simulink model "Lazoabierto_ruido"  (R2021b)
settings: Solver=VariableStepAuto  StartTime=0.0  StopTime=500  RelTol=1e-3
libraries: fl_lib x15, nesl_utility x9, simulink x3, sh_lib x3
settings Model: Creator=sebas  LastModifiedBy=sebas

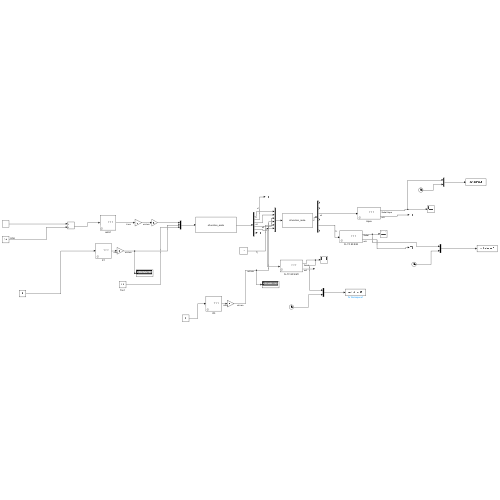
[thumbnail: Simulink's stored preview of the top-level diagram]
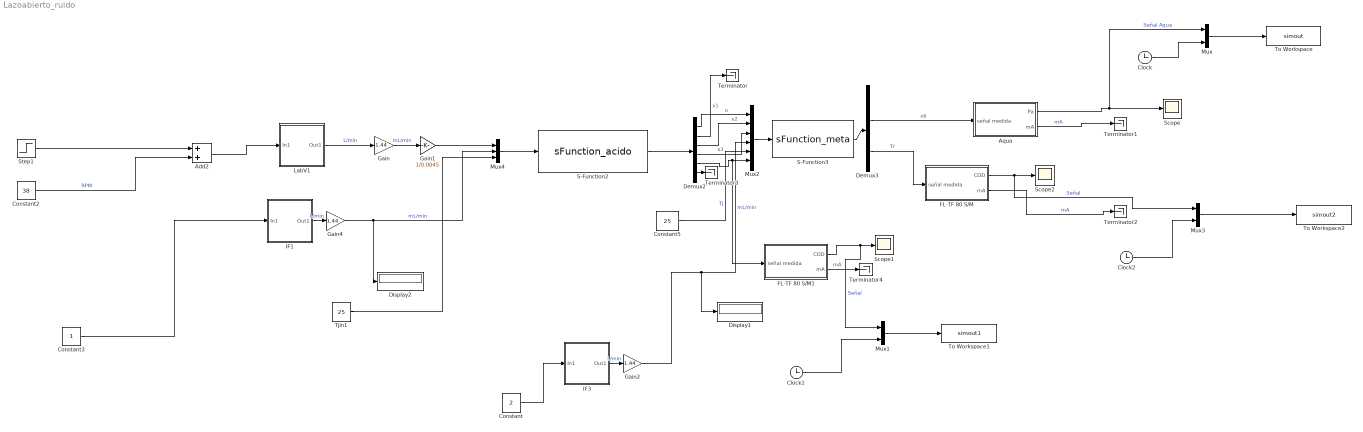
== system Lazoabierto_ruido ==
  Add2 : Sum
  Aqua : Subsystem  mask{To=0.01, d=0, DS=2.5, Ks=0.0056, Tau=1, yo=0, Vi=10}
      mask prompts: To "Tiempo de muestreo (s)"; d "Retardo (s)"; DS "Desviacion estandar (mg/L)"; Ks "Sensibilidad (mA/mg/L)"; Tau "Constante de tiempo (s)"; yo "Sesgo (mg/L)"; Vi "Valor inicial (mg/L)"
      mask init:
      | NP=To*DS*DS;
      mask Display: image(imread('sensor3.png'))
  Clock : Clock
  Clock1 : Clock
  Clock2 : Clock
  Constant : Constant  Value=2
  Constant2 : Constant  Value=38
  Constant3 : Constant
  Constant5 : Constant  Value=25
  Demux2 : Demux  Outputs=6
  Demux3 : Demux  Outputs=6
  Display1 : Display
  Display2 : Display
  FL-TF 80 S/M : Subsystem  mask{To=0.001, d=0, DS=0.15, Ks=0.175, Tau=0.0000667, yo=0, Vi=65}
      mask prompts: To "Tiempo de muestreo (s)"; d "Retardo (s)"; DS "Desviacion estandar (C°)"; Ks "Sensibilidad (mA/C°)"; Tau "Constante de tiempo (s)"; yo "Sesgo (C°)"; Vi "Valor inicial (C°)"
      mask init:
      | NP=To*DS*DS;
      mask Display: image(imread('sensor5.png'))
  FL-TF 80 S/M1 : Subsystem  mask{To=0.001, d=0, DS=0.15, Ks=0.175, Tau=0.0000667, yo=0, Vi=37}
      mask prompts: To "Tiempo de muestreo (s)"; d "Retardo (s)"; DS "Desviacion estandar (C°)"; Ks "Sensibilidad (mA/C°)"; Tau "Constante de tiempo (s)"; yo "Sesgo (C°)"; Vi "Valor inicial (C°)"
      mask init:
      | NP=To*DS*DS;
      mask Display: image(imread('sensor5.png'))
  Gain : Gain  Gain=1.44
  Gain1 : Gain  Gain=1/0.0045
  Gain2 : Gain  Gain=1.44
  Gain4 : Gain  Gain=1.44
  IF1 : Subsystem  mask{D=0.00955414, MaxRPM=350, MaxLPM=4.34, OutP=0.1, FluidDens=997, KinemVisc=0.893e-6, BulkMod=2.2e+9}
      mask prompts: D "Displacement [L/rev]"; MaxRPM "RPM Máximas [RPM]"; MaxLPM "Caudal Máximo [L/min]"; OutP "Presión de Salida [MPa]"; FluidDens "Densidad del Fluido [kg/m^3]"; KinemVisc "Viscosidad Cinemática del Fluido [m^2/s]"; BulkMod "Modulo de Compresibilidad del Fluido [Pa]"
      mask help:
      | Simulación de una Bomba Peristáltica utilizando el paquete Simscape (puede entrar en el subsistema para ver en base a que bloques se construyó).
      |
      | El principal parámetro es el Displacement, que representa cuánto aumenta el flujo de la bomba medido en Litros por Minuto [L/min] según el aumento unitario de Revoluciones por Minuto [RPM].
      |
      | El input de este bloque es una fuente de revoluciones en unidades de RPM, el cual entrega un output de caudal en L/min.
      |
      | El valor del Displacement no puede superar su valor máximo según los parámetros entregados de la bomba.
      mask Display:
      | image('bomba3.png'); % Use "Edit Image" on toolstrip to change.
      | % Bloque creado por Tomás Pröschle Donoso - DCP 2020-2
  IF3 : Subsystem  mask{D=0.00955414, MaxRPM=350, MaxLPM=4.34, OutP=0.1, FluidDens=997, KinemVisc=0.893e-6, BulkMod=2.2e+9}
      mask prompts: D "Displacement [L/rev]"; MaxRPM "RPM Máximas [RPM]"; MaxLPM "Caudal Máximo [L/min]"; OutP "Presión de Salida [MPa]"; FluidDens "Densidad del Fluido [kg/m^3]"; KinemVisc "Viscosidad Cinemática del Fluido [m^2/s]"; BulkMod "Modulo de Compresibilidad del Fluido [Pa]"
      mask help:
      | Simulación de una Bomba Peristáltica utilizando el paquete Simscape (puede entrar en el subsistema para ver en base a que bloques se construyó).
      |
      | El principal parámetro es el Displacement, que representa cuánto aumenta el flujo de la bomba medido en Litros por Minuto [L/min] según el aumento unitario de Revoluciones por Minuto [RPM].
      |
      | El input de este bloque es una fuente de revoluciones en unidades de RPM, el cual entrega un output de caudal en L/min.
      |
      | El valor del Displacement no puede superar su valor máximo según los parámetros entregados de la bomba.
      mask Display:
      | image('bomba3.png'); % Use "Edit Image" on toolstrip to change.
      | % Bloque creado por Tomás Pröschle Donoso - DCP 2020-2
  LabV1 : Subsystem  mask{D=0.00001333, MaxRPM=150, MaxLPM=0.57, OutP=0.1, FluidDens=997, KinemVisc=0.893e-6, BulkMod=2.2e+9}
      mask prompts: D "Displacement [L/rev]"; MaxRPM "RPM Máximas [RPM]"; MaxLPM "Caudal Máximo [L/min]"; OutP "Presión de Salida [MPa]"; FluidDens "Densidad del Fluido [kg/m^3]"; KinemVisc "Viscosidad Cinemática del Fluido [m^2/s]"; BulkMod "Modulo de Compresibilidad del Fluido [Pa]"
      mask help:
      | Simulación de una Bomba Peristáltica utilizando el paquete Simscape (puede entrar en el subsistema para ver en base a que bloques se construyó).
      |
      | El principal parámetro es el Displacement, que representa cuánto aumenta el flujo de la bomba medido en Litros por Minuto [L/min] según el aumento unitario de Revoluciones por Minuto [RPM].
      |
      | El input de este bloque es una fuente de revoluciones en unidades de RPM, el cual entrega un output de caudal en L/min.
      |
      | El valor del Displacement no puede superar su valor máximo según los parámetros entregados de la bomba.
      mask Display:
      | image('bomba1.png'); % Use "Edit Image" on toolstrip to change.
      | % Bloque creado por Tomás Pröschle Donoso - DCP 2020-2
  Mux : Mux  Inputs=2
  Mux1 : Mux  Inputs=2
  Mux2 : Mux  Inputs=6
  Mux3 : Mux  Inputs=2
  Mux4 : Mux  Inputs=3
  S-Function2 : S-Function  FunctionName=sFunction_acido  SFunctionDeploymentMode=off  EnableBusSupport=off
  S-Function3 : S-Function  FunctionName=sFunction_meta  SFunctionDeploymentMode=off  EnableBusSupport=off
  Scope : Scope
  Scope1 : Scope
  Scope2 : Scope
  Step1 : Step  Time=100  After=100  SampleTime=0
  Terminator{,1..4} (5 alike) : Terminator
  Tjin1 : Constant  Value=25
  To Workspace : ToWorkspace  VariableName=simout  SampleTime=-1
  To Workspace1 : ToWorkspace  VariableName=simout1  SampleTime=-1
  To Workspace2 : ToWorkspace  VariableName=simout2  SampleTime=-1
  wires:
  Tjin1/1 -> Mux4/3
  Demux3/5 -> FL-TF 80 S/M/1(señal medida)  "Tr"
  Demux2/3 -> Mux2/2  "x2"
  S-Function3/1 -> Demux3/1
  Mux2/1 -> S-Function3/1
  Mux4/1 -> S-Function2/1
  Demux2/6 -> Terminator3/1
  Constant5/1 -> Mux2/5  "Tj"
  Demux2/2 -> Terminator/1  "x1"
  Demux2/4 -> Mux2/3  "x3"
  Demux2/1 -> Mux2/1  "u"
  Demux3/3 -> Aqua/1(señal medida)  "x6"
  Demux2/5 -> FL-TF 80 S/M1/1(señal medida), Mux2/6
  S-Function2/1 -> Demux2/1
  Gain1/1 -> Mux4/1
  LabV1/1(Out1) -> Gain/1  "L/min"
  Constant2/1 -> Add2/2  "RPM"
  Gain/1 -> Gain1/1  "mL/min"
  Gain4/1 -> Display2/1, Mux4/2  "mL/min"
  Constant/1 -> IF3/1(In1)
  Aqua/2(mA) -> Terminator1/1  "mA"
  Aqua/1(Pa) -> Mux/1, Scope/1  "Señal Aqua"
  FL-TF 80 S/M/2(mA) -> Terminator2/1  "mA"
  FL-TF 80 S/M/1(COD) -> Mux3/1, Scope2/1  "Señal"
  FL-TF 80 S/M1/2(mA) -> Terminator4/1  "mA"
  FL-TF 80 S/M1/1(COD) -> Mux1/1, Scope1/1  "Señal"
  Gain2/1 -> Display1/1, Mux2/4  "mL/min"
  IF3/1(Out1) -> Gain2/1  "L/min"
  IF1/1(Out1) -> Gain4/1  "L/min"
  Step1/1 -> Add2/1
  Constant3/1 -> IF1/1(In1)
  Add2/1 -> LabV1/1(In1)
  Clock/1 -> Mux/2
  Mux/1 -> To Workspace/1
  Clock1/1 -> Mux1/2
  Mux1/1 -> To Workspace1/1
  Clock2/1 -> Mux3/2
  Mux3/1 -> To Workspace2/1

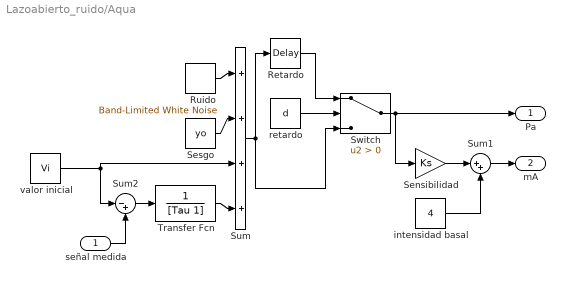
== system Lazoabierto_ruido/Aqua ==
  señal medida : Inport
  Retardo : TransportDelay  DelayTime=d
  Ruido : simulink/Sources/Band-Limited White Noise  Cov=[NP]  Ts=To  seed=[23341]
  Sensibilidad : Gain  Gain=Ks
  Sesgo : Constant  Value=yo
  Sum : Sum  Inputs=|++++  SaturateOnIntegerOverflow=on
  Sum1 : Sum  Inputs=|++
  Sum2 : Sum  Inputs=|-+
  Switch : Switch  Criteria=u2 > Threshold
  Transfer Fcn : TransferFcn  Denominator=[Tau 1]
  intensidad basal : Constant  Value=4
  retardo : Constant  Value=d
  valor inicial : Constant  Value=Vi
  Pa : Outport
  mA : Outport  Port=2
  wires:
  Sensibilidad/1 -> Sum1/1
  Sum1/1 -> mA/1
  intensidad basal/1 -> Sum1/2
  retardo/1 -> Switch/2
  Sum/1 -> Retardo/1, Switch/3
  Retardo/1 -> Switch/1
  Switch/1 -> Pa/1, Sensibilidad/1
  Sesgo/1 -> Sum/2
  Ruido/1 -> Sum/1
  Transfer Fcn/1 -> Sum/4
  Sum2/1 -> Transfer Fcn/1
  señal medida/1 -> Sum2/2
  valor inicial/1 -> Sum/3, Sum2/1

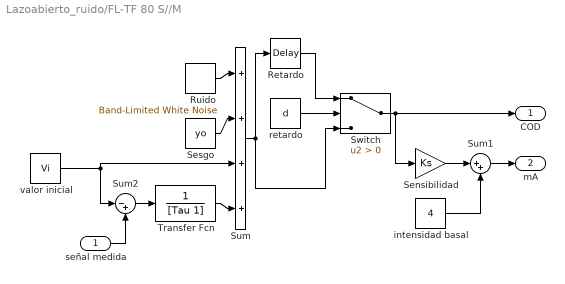
== system Lazoabierto_ruido/FL-TF 80 S//M ==
  señal medida : Inport
  Retardo : TransportDelay  DelayTime=d
  Ruido : simulink/Sources/Band-Limited White Noise  Cov=[NP]  Ts=To  seed=[23341]
  Sensibilidad : Gain  Gain=Ks
  Sesgo : Constant  Value=yo
  Sum : Sum  Inputs=|++++  SaturateOnIntegerOverflow=on
  Sum1 : Sum  Inputs=|++
  Sum2 : Sum  Inputs=|-+
  Switch : Switch  Criteria=u2 > Threshold
  Transfer Fcn : TransferFcn  Denominator=[Tau 1]
  intensidad basal : Constant  Value=4
  retardo : Constant  Value=d
  valor inicial : Constant  Value=Vi
  COD : Outport
  mA : Outport  Port=2
  wires:
  Sensibilidad/1 -> Sum1/1
  Sum1/1 -> mA/1
  intensidad basal/1 -> Sum1/2
  retardo/1 -> Switch/2
  Sum/1 -> Retardo/1, Switch/3
  Retardo/1 -> Switch/1
  Switch/1 -> COD/1, Sensibilidad/1
  Sesgo/1 -> Sum/2
  Ruido/1 -> Sum/1
  Transfer Fcn/1 -> Sum/4
  Sum2/1 -> Transfer Fcn/1
  señal medida/1 -> Sum2/2
  valor inicial/1 -> Sum/3, Sum2/1

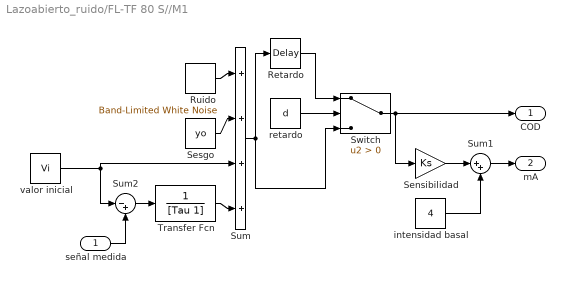
== system Lazoabierto_ruido/FL-TF 80 S//M1 ==
  señal medida : Inport
  Retardo : TransportDelay  DelayTime=d
  Ruido : simulink/Sources/Band-Limited White Noise  Cov=[NP]  Ts=To  seed=[23341]
  Sensibilidad : Gain  Gain=Ks
  Sesgo : Constant  Value=yo
  Sum : Sum  Inputs=|++++  SaturateOnIntegerOverflow=on
  Sum1 : Sum  Inputs=|++
  Sum2 : Sum  Inputs=|-+
  Switch : Switch  Criteria=u2 > Threshold
  Transfer Fcn : TransferFcn  Denominator=[Tau 1]
  intensidad basal : Constant  Value=4
  retardo : Constant  Value=d
  valor inicial : Constant  Value=Vi
  COD : Outport
  mA : Outport  Port=2
  wires:
  Sensibilidad/1 -> Sum1/1
  Sum1/1 -> mA/1
  intensidad basal/1 -> Sum1/2
  retardo/1 -> Switch/2
  Sum/1 -> Retardo/1, Switch/3
  Retardo/1 -> Switch/1
  Switch/1 -> COD/1, Sensibilidad/1
  Sesgo/1 -> Sum/2
  Ruido/1 -> Sum/1
  Transfer Fcn/1 -> Sum/4
  Sum2/1 -> Transfer Fcn/1
  señal medida/1 -> Sum2/2
  valor inicial/1 -> Sum/3, Sum2/1

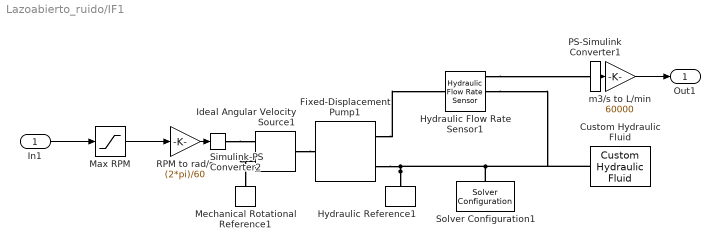
== system Lazoabierto_ruido/IF1 ==
  In1 : Inport
  Custom Hydraulic Fluid : fl_lib/Hydraulic/Hydraulic Utilities/Custom Hydraulic Fluid  density=FluidDens kg/m^3  viscosity_kin=KinemVisc m^2/s  bulk=BulkMod Pa  alpha=0  range_error=2
      settings: SourceProductBaseCode=SS  InternalSimscapePortConfiguration="{\"Bottom\":[],\"Left\":[],\"Right\":[{\"id\":\"G\",\"label\":\"\",\"type\":\"foundation.hydraulic.hydraulic\"}],\"Top\":[]}"
  Fixed-Displacement Pump1 : sh_lib/Pumps and Motors/Fixed-Displacement Pump  D=D l/rev  loss_spec=1  w_nominal=MaxRPM rpm  pr_nominal=OutP MPa  visc_nominal=KinemVisc m^2/s  dens_nominal=FluidDens kg/m^3  efficiency_vol=1  no_load_torque=0 N*m  torque_pressure_coeff=0 N*m/Pa  p_diff_eff_TLU=[100000, 1000000, 2000000] Pa  omega_eff_TLU=[25, 50, 100, 200, 300, 400] rad/s  vol_eff_TLU=[.816, .908, .954, .977, .981, .984; .325, .663, .831, .916, .925, .946; .137, .568, .78, .892, .893, .91]  mech_eff_TLU=[.996, .996, .996, .996, .996, .996; .988, .989, .989, .989, .989, .99; .981, .981, .982, .982, .983, .984]  p_diff_loss_TLU=[100000, 1000000, 2000000] Pa  omega_loss_TLU=[25, 50, 100, 200, 300, 400] rad/s  vol_loss_TLU=[.023, .023, .023, .023, .0285, .032; .0844, .0842, .0845, .084, .1125, .108; .1079, .108, .11, .108, .1605, .18] * 1e-3 m^3/s  mech_loss_TLU=[.002, .002, .002, .002, .002, .002; .0607, .0556, .0556, .0556, .0556, .0505; .1937, .1937, .1833, .1833, .1729, .1626] N*m  pressure_threshold=1e5 Pa  omega_threshold=10 rad/s  quadrant_check=0  pressure_check=0  min_valid_pressure=0 Pa  vol_eff_min=1e-3  vol_eff_max=1  mech_eff_min=1e-3  mech_eff_max=1
      settings: SourceProductBaseCode=SH  InternalSimscapePortConfiguration="{\"Bottom\":[],\"Left\":[{\"id\":\"S\",\"label\":\"S\",\"type\":\"foundation.mechanical.rotational.rotational\"}],\"Right\":[{\"id\":\"P\",\"label\":\"P\",\"type\":\"foundation.hydraulic.hydraulic\"},{\"id\":\"T\",\"label\":\"T\",\"type\":\"foundation.hydraulic.hydraulic\"}],\"Top\":[]}"
  Hydraulic Flow Rate Sensor1 : fl_lib/Hydraulic/Hydraulic Sensors/Hydraulic Flow Rate Sensor
  Hydraulic Reference1 : fl_lib/Hydraulic/Hydraulic Elements/Hydraulic Reference
  Ideal Angular Velocity Source1 : fl_lib/Mechanical/Mechanical Sources/Ideal Angular Velocity Source
  Max RPM : Saturate  UpperLimit=600  LowerLimit=0
  Mechanical Rotational Reference1 : fl_lib/Mechanical/Rotational Elements/Mechanical Rotational Reference
  PS-Simulink Converter1 : nesl_utility/PS-Simulink Converter  PhysicalDomain=network_engine_domain  SubClassName=ps_output  LeftPortType=input  RightPortType=output  PseudoPeriodic=off  Frequencies=[]  Unit=inherit  AffineConversion=off
      settings: SourceProductBaseCode=PW,SS
  RPM to rad/s : Gain  Gain=(2*pi)/60
  Simulink-PS Converter2 : nesl_utility/Simulink-PS Converter  PhysicalDomain=network_engine_domain  SubClassName=ps_input  LeftPortType=input  RightPortType=output  PseudoPeriodic=off  Frequencies=[]  NoiseDistribution=none  NoiseParameters=[]  Unit=1  AffineConversion=off  FilteringAndDerivatives=provide  SimscapeFilterOrder=1  InputFilterTimeConstant=0.001  UdotUserProvided=0
      settings: SourceProductBaseCode=PW,SS
  Solver Configuration1 : nesl_utility/Solver Configuration  PhysicalDomain=network_engine_domain  SubClassName=solver  LeftPortType=input  RightPortType=generic  Tones=[]  Harmonics=[]  SimulateNoise=off  Profile=off  UseLocalSampling=off  EnableSwitchedLinearOptims=on  FrequencyDomain=off  UseCCode=off  RelTol=0.001  AbsTol=1e-06  MinStep=1e-09  ToWorkspace=off  RevertToSquareIcSolve=off  NumHomotopyIterations=100  PhasorMode=off  PhasorModeNumHarmonics=1  DoDC=off  ResidualTolerance=1e-09  UseLocalSolver=off  LocalSolverChoice=NE_BACKWARD_EULER_ADVANCER  LocalSolverSampleTime=0.001  DoFixedCost=off  MaxNonlinIter=3  MaxModeIter=2  ComputeImpulses=off  ImpulseIterations=2  LinearAlgebra=auto  EquationFormulation=NE_TIME_EF  DelaysMemoryBudget=1024  AutomaticFiltering=on  FilteringTimeConstant=0.001  PartitionStorageMethod=AS_NEEDED  PartitionMemoryBudget=1024  PartitionMethod=ROBUST
      settings: SourceProductBaseCode=PW,SS
  m3/s to L/min : Gain  Gain=60000
  Out1 : Outport
  wires:
  RPM to rad/s/1 -> Simulink-PS Converter2/1
  PS-Simulink Converter1/1 -> m3/s to L/min/1
  In1/1 -> Max RPM/1
  m3/s to L/min/1 -> Out1/1
  Max RPM/1 -> RPM to rad/s/1
  connections:
  Hydraulic Reference1/LConn1 -- Custom Hydraulic Fluid/RConn1 -- Hydraulic Flow Rate Sensor1/RConn2 -- Solver Configuration1/RConn1 -- Fixed-Displacement Pump1/RConn2
  Simulink-PS Converter2/RConn1 -- Ideal Angular Velocity Source1/RConn1
  Ideal Angular Velocity Source1/RConn2 -- Mechanical Rotational Reference1/LConn1
  Hydraulic Flow Rate Sensor1/RConn1 -- PS-Simulink Converter1/LConn1
  Fixed-Displacement Pump1/RConn1 -- Hydraulic Flow Rate Sensor1/LConn1
  Ideal Angular Velocity Source1/LConn1 -- Fixed-Displacement Pump1/LConn1

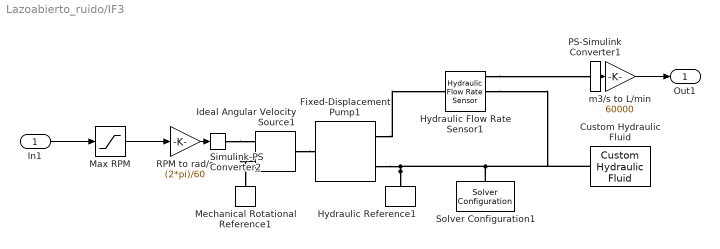
== system Lazoabierto_ruido/IF3 ==
  In1 : Inport
  Custom Hydraulic Fluid : fl_lib/Hydraulic/Hydraulic Utilities/Custom Hydraulic Fluid  density=FluidDens kg/m^3  viscosity_kin=KinemVisc m^2/s  bulk=BulkMod Pa  alpha=0  range_error=2
      settings: SourceProductBaseCode=SS  InternalSimscapePortConfiguration="{\"Bottom\":[],\"Left\":[],\"Right\":[{\"id\":\"G\",\"label\":\"\",\"type\":\"foundation.hydraulic.hydraulic\"}],\"Top\":[]}"
  Fixed-Displacement Pump1 : sh_lib/Pumps and Motors/Fixed-Displacement Pump  D=D l/rev  loss_spec=1  w_nominal=MaxRPM rpm  pr_nominal=OutP MPa  visc_nominal=KinemVisc m^2/s  dens_nominal=FluidDens kg/m^3  efficiency_vol=1  no_load_torque=0 N*m  torque_pressure_coeff=0 N*m/Pa  p_diff_eff_TLU=[100000, 1000000, 2000000] Pa  omega_eff_TLU=[25, 50, 100, 200, 300, 400] rad/s  vol_eff_TLU=[.816, .908, .954, .977, .981, .984; .325, .663, .831, .916, .925, .946; .137, .568, .78, .892, .893, .91]  mech_eff_TLU=[.996, .996, .996, .996, .996, .996; .988, .989, .989, .989, .989, .99; .981, .981, .982, .982, .983, .984]  p_diff_loss_TLU=[100000, 1000000, 2000000] Pa  omega_loss_TLU=[25, 50, 100, 200, 300, 400] rad/s  vol_loss_TLU=[.023, .023, .023, .023, .0285, .032; .0844, .0842, .0845, .084, .1125, .108; .1079, .108, .11, .108, .1605, .18] * 1e-3 m^3/s  mech_loss_TLU=[.002, .002, .002, .002, .002, .002; .0607, .0556, .0556, .0556, .0556, .0505; .1937, .1937, .1833, .1833, .1729, .1626] N*m  pressure_threshold=1e5 Pa  omega_threshold=10 rad/s  quadrant_check=0  pressure_check=0  min_valid_pressure=0 Pa  vol_eff_min=1e-3  vol_eff_max=1  mech_eff_min=1e-3  mech_eff_max=1
      settings: SourceProductBaseCode=SH  InternalSimscapePortConfiguration="{\"Bottom\":[],\"Left\":[{\"id\":\"S\",\"label\":\"S\",\"type\":\"foundation.mechanical.rotational.rotational\"}],\"Right\":[{\"id\":\"P\",\"label\":\"P\",\"type\":\"foundation.hydraulic.hydraulic\"},{\"id\":\"T\",\"label\":\"T\",\"type\":\"foundation.hydraulic.hydraulic\"}],\"Top\":[]}"
  Hydraulic Flow Rate Sensor1 : fl_lib/Hydraulic/Hydraulic Sensors/Hydraulic Flow Rate Sensor
  Hydraulic Reference1 : fl_lib/Hydraulic/Hydraulic Elements/Hydraulic Reference
  Ideal Angular Velocity Source1 : fl_lib/Mechanical/Mechanical Sources/Ideal Angular Velocity Source
  Max RPM : Saturate  UpperLimit=600  LowerLimit=0
  Mechanical Rotational Reference1 : fl_lib/Mechanical/Rotational Elements/Mechanical Rotational Reference
  PS-Simulink Converter1 : nesl_utility/PS-Simulink Converter  PhysicalDomain=network_engine_domain  SubClassName=ps_output  LeftPortType=input  RightPortType=output  PseudoPeriodic=off  Frequencies=[]  Unit=inherit  AffineConversion=off
      settings: SourceProductBaseCode=PW,SS
  RPM to rad/s : Gain  Gain=(2*pi)/60
  Simulink-PS Converter2 : nesl_utility/Simulink-PS Converter  PhysicalDomain=network_engine_domain  SubClassName=ps_input  LeftPortType=input  RightPortType=output  PseudoPeriodic=off  Frequencies=[]  NoiseDistribution=none  NoiseParameters=[]  Unit=1  AffineConversion=off  FilteringAndDerivatives=provide  SimscapeFilterOrder=1  InputFilterTimeConstant=0.001  UdotUserProvided=0
      settings: SourceProductBaseCode=PW,SS
  Solver Configuration1 : nesl_utility/Solver Configuration  PhysicalDomain=network_engine_domain  SubClassName=solver  LeftPortType=input  RightPortType=generic  Tones=[]  Harmonics=[]  SimulateNoise=off  Profile=off  UseLocalSampling=off  EnableSwitchedLinearOptims=on  FrequencyDomain=off  UseCCode=off  RelTol=0.001  AbsTol=1e-06  MinStep=1e-09  ToWorkspace=off  RevertToSquareIcSolve=off  NumHomotopyIterations=100  PhasorMode=off  PhasorModeNumHarmonics=1  DoDC=off  ResidualTolerance=1e-09  UseLocalSolver=off  LocalSolverChoice=NE_BACKWARD_EULER_ADVANCER  LocalSolverSampleTime=0.001  DoFixedCost=off  MaxNonlinIter=3  MaxModeIter=2  ComputeImpulses=off  ImpulseIterations=2  LinearAlgebra=auto  EquationFormulation=NE_TIME_EF  DelaysMemoryBudget=1024  AutomaticFiltering=on  FilteringTimeConstant=0.001  PartitionStorageMethod=AS_NEEDED  PartitionMemoryBudget=1024  PartitionMethod=ROBUST
      settings: SourceProductBaseCode=PW,SS
  m3/s to L/min : Gain  Gain=60000
  Out1 : Outport
  wires:
  RPM to rad/s/1 -> Simulink-PS Converter2/1
  PS-Simulink Converter1/1 -> m3/s to L/min/1
  In1/1 -> Max RPM/1
  m3/s to L/min/1 -> Out1/1
  Max RPM/1 -> RPM to rad/s/1
  connections:
  Hydraulic Reference1/LConn1 -- Custom Hydraulic Fluid/RConn1 -- Hydraulic Flow Rate Sensor1/RConn2 -- Solver Configuration1/RConn1 -- Fixed-Displacement Pump1/RConn2
  Simulink-PS Converter2/RConn1 -- Ideal Angular Velocity Source1/RConn1
  Ideal Angular Velocity Source1/RConn2 -- Mechanical Rotational Reference1/LConn1
  Hydraulic Flow Rate Sensor1/RConn1 -- PS-Simulink Converter1/LConn1
  Fixed-Displacement Pump1/RConn1 -- Hydraulic Flow Rate Sensor1/LConn1
  Ideal Angular Velocity Source1/LConn1 -- Fixed-Displacement Pump1/LConn1

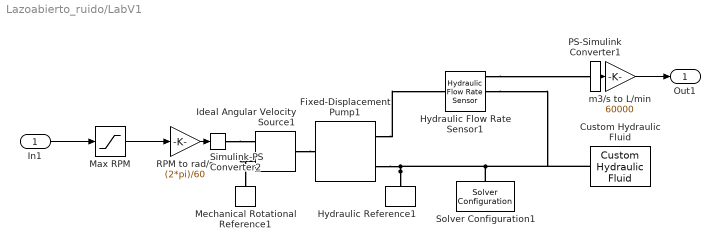
== system Lazoabierto_ruido/LabV1 ==
  In1 : Inport
  Custom Hydraulic Fluid : fl_lib/Hydraulic/Hydraulic Utilities/Custom Hydraulic Fluid  density=FluidDens kg/m^3  viscosity_kin=KinemVisc m^2/s  bulk=BulkMod Pa  alpha=0  range_error=2
      settings: SourceProductBaseCode=SS  InternalSimscapePortConfiguration="{\"Bottom\":[],\"Left\":[],\"Right\":[{\"id\":\"G\",\"label\":\"\",\"type\":\"foundation.hydraulic.hydraulic\"}],\"Top\":[]}"
  Fixed-Displacement Pump1 : sh_lib/Pumps and Motors/Fixed-Displacement Pump  D=D l/rev  loss_spec=1  w_nominal=MaxRPM rpm  pr_nominal=OutP MPa  visc_nominal=KinemVisc m^2/s  dens_nominal=FluidDens kg/m^3  efficiency_vol=1  no_load_torque=0 N*m  torque_pressure_coeff=0 N*m/Pa  p_diff_eff_TLU=[100000, 1000000, 2000000] Pa  omega_eff_TLU=[25, 50, 100, 200, 300, 400] rad/s  vol_eff_TLU=[.816, .908, .954, .977, .981, .984; .325, .663, .831, .916, .925, .946; .137, .568, .78, .892, .893, .91]  mech_eff_TLU=[.996, .996, .996, .996, .996, .996; .988, .989, .989, .989, .989, .99; .981, .981, .982, .982, .983, .984]  p_diff_loss_TLU=[100000, 1000000, 2000000] Pa  omega_loss_TLU=[25, 50, 100, 200, 300, 400] rad/s  vol_loss_TLU=[.023, .023, .023, .023, .0285, .032; .0844, .0842, .0845, .084, .1125, .108; .1079, .108, .11, .108, .1605, .18] * 1e-3 m^3/s  mech_loss_TLU=[.002, .002, .002, .002, .002, .002; .0607, .0556, .0556, .0556, .0556, .0505; .1937, .1937, .1833, .1833, .1729, .1626] N*m  pressure_threshold=1e5 Pa  omega_threshold=10 rad/s  quadrant_check=0  pressure_check=0  min_valid_pressure=0 Pa  vol_eff_min=1e-3  vol_eff_max=1  mech_eff_min=1e-3  mech_eff_max=1
      settings: SourceProductBaseCode=SH  InternalSimscapePortConfiguration="{\"Bottom\":[],\"Left\":[{\"id\":\"S\",\"label\":\"S\",\"type\":\"foundation.mechanical.rotational.rotational\"}],\"Right\":[{\"id\":\"P\",\"label\":\"P\",\"type\":\"foundation.hydraulic.hydraulic\"},{\"id\":\"T\",\"label\":\"T\",\"type\":\"foundation.hydraulic.hydraulic\"}],\"Top\":[]}"
  Hydraulic Flow Rate Sensor1 : fl_lib/Hydraulic/Hydraulic Sensors/Hydraulic Flow Rate Sensor
  Hydraulic Reference1 : fl_lib/Hydraulic/Hydraulic Elements/Hydraulic Reference
  Ideal Angular Velocity Source1 : fl_lib/Mechanical/Mechanical Sources/Ideal Angular Velocity Source
  Max RPM : Saturate  UpperLimit=600  LowerLimit=0
  Mechanical Rotational Reference1 : fl_lib/Mechanical/Rotational Elements/Mechanical Rotational Reference
  PS-Simulink Converter1 : nesl_utility/PS-Simulink Converter  PhysicalDomain=network_engine_domain  SubClassName=ps_output  LeftPortType=input  RightPortType=output  PseudoPeriodic=off  Frequencies=[]  Unit=inherit  AffineConversion=off
      settings: SourceProductBaseCode=PW,SS
  RPM to rad/s : Gain  Gain=(2*pi)/60
  Simulink-PS Converter2 : nesl_utility/Simulink-PS Converter  PhysicalDomain=network_engine_domain  SubClassName=ps_input  LeftPortType=input  RightPortType=output  PseudoPeriodic=off  Frequencies=[]  NoiseDistribution=none  NoiseParameters=[]  Unit=1  AffineConversion=off  FilteringAndDerivatives=provide  SimscapeFilterOrder=1  InputFilterTimeConstant=0.001  UdotUserProvided=0
      settings: SourceProductBaseCode=PW,SS
  Solver Configuration1 : nesl_utility/Solver Configuration  PhysicalDomain=network_engine_domain  SubClassName=solver  LeftPortType=input  RightPortType=generic  Tones=[]  Harmonics=[]  SimulateNoise=off  Profile=off  UseLocalSampling=off  EnableSwitchedLinearOptims=on  FrequencyDomain=off  UseCCode=off  RelTol=0.001  AbsTol=1e-06  MinStep=1e-09  ToWorkspace=off  RevertToSquareIcSolve=off  NumHomotopyIterations=100  PhasorMode=off  PhasorModeNumHarmonics=1  DoDC=off  ResidualTolerance=1e-09  UseLocalSolver=off  LocalSolverChoice=NE_BACKWARD_EULER_ADVANCER  LocalSolverSampleTime=0.001  DoFixedCost=off  MaxNonlinIter=3  MaxModeIter=2  ComputeImpulses=off  ImpulseIterations=2  LinearAlgebra=auto  EquationFormulation=NE_TIME_EF  DelaysMemoryBudget=1024  AutomaticFiltering=on  FilteringTimeConstant=0.001  PartitionStorageMethod=AS_NEEDED  PartitionMemoryBudget=1024  PartitionMethod=ROBUST
      settings: SourceProductBaseCode=PW,SS
  m3/s to L/min : Gain  Gain=60000
  Out1 : Outport
  wires:
  RPM to rad/s/1 -> Simulink-PS Converter2/1
  PS-Simulink Converter1/1 -> m3/s to L/min/1
  In1/1 -> Max RPM/1
  m3/s to L/min/1 -> Out1/1
  Max RPM/1 -> RPM to rad/s/1
  connections:
  Hydraulic Reference1/LConn1 -- Custom Hydraulic Fluid/RConn1 -- Hydraulic Flow Rate Sensor1/RConn2 -- Solver Configuration1/RConn1 -- Fixed-Displacement Pump1/RConn2
  Simulink-PS Converter2/RConn1 -- Ideal Angular Velocity Source1/RConn1
  Ideal Angular Velocity Source1/RConn2 -- Mechanical Rotational Reference1/LConn1
  Hydraulic Flow Rate Sensor1/RConn1 -- PS-Simulink Converter1/LConn1
  Fixed-Displacement Pump1/RConn1 -- Hydraulic Flow Rate Sensor1/LConn1
  Ideal Angular Velocity Source1/LConn1 -- Fixed-Displacement Pump1/LConn1
